simulink model "Exercise42"  (R2016a)
settings: Solver=VariableStepAuto  StartTime=0.0  StopTime=0.200  RelTol=1e-3
undefined symbols (not defined in the file): f, J, K, ke, kt, L, Mb, R
settings Model: Creator=Ramiro  LastModifiedBy=Ramiro

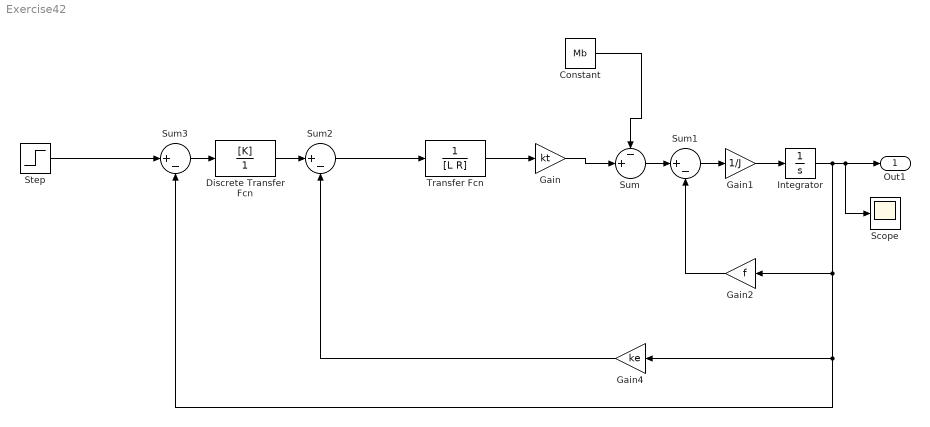
== system Exercise42 ==
  Constant : Constant  Value=Mb
  Discrete Transfer Fcn : DiscreteTransferFcn  Numerator=[K]  Denominator=[1]  SampleTime=0.005
  Gain : Gain  Gain=kt
  Gain1 : Gain  Gain=1/J
  Gain2 : Gain  Gain=f
  Gain4 : Gain  Gain=ke
  Integrator : Integrator
  Scope : Scope
  Step : Step  Time=0  After=1/0.86  SampleTime=0
  Sum : Sum  Inputs=-+|
  Sum1 : Sum  Inputs=|+-
  Sum2 : Sum  Inputs=|+-
  Sum3 : Sum  Inputs=|+-
  Transfer Fcn : TransferFcn  Denominator=[L R]
  Out1 : Outport
  wires:
  Gain/1 -> Sum/2
  Constant/1 -> Sum/1
  Sum/1 -> Sum1/1
  Sum1/1 -> Gain1/1
  Gain2/1 -> Sum1/2
  Transfer Fcn/1 -> Gain/1
  Sum2/1 -> Transfer Fcn/1
  Gain1/1 -> Integrator/1
  Gain4/1 -> Sum2/2
  Integrator/1 -> Out1/1, Scope/1, Gain4/1, Sum3/2, Gain2/1
  Discrete Transfer Fcn/1 -> Sum2/1
  Step/1 -> Sum3/1
  Sum3/1 -> Discrete Transfer Fcn/1
